simulink model "Lab_1b_sim"  (R2017a)
settings: Solver=VariableStepAuto  StartTime=0.0  StopTime=1.0  RelTol=1e-3
values from neighbouring files (symbols this model uses):
  alpha = 26.66    [Lab_1.m]    (also in Lab_2.m)
  alpha_p = 32.7345    [Lab_1.m]    (also in Lab_2.m)
  beta = 133.33    [Lab_1.m]    (also in Lab_2.m)
  K = f*(alpha_p.^2)/(4*beta)    [Lab_1.m]    (also in Lab_2.m)
  Kf = alpha_p/2    (= 16.36725)    [Lab_1.m]    (also in Lab_2.m)
settings Model: Creator=njohnson  LastModifiedBy=njohnson

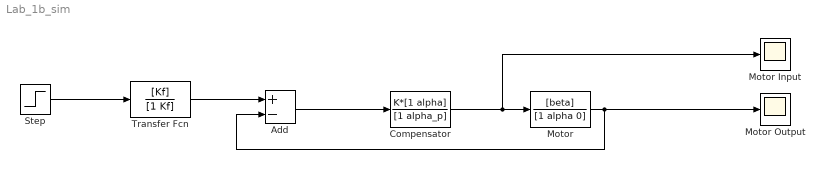
== system Lab_1b_sim ==
  Add : Sum  Inputs=+-
  "Compensator " : TransferFcn  Numerator=K*[1 alpha]  Denominator=[1 alpha_p]
  "Motor " : TransferFcn  Numerator=[beta]  Denominator=[1 alpha 0]
  Motor Input : Scope
  Motor Output : Scope
  Step : Step  Time=0  After=3  SampleTime=0
  Transfer Fcn : TransferFcn  Numerator=[Kf]  Denominator=[1 Kf]
  wires:
  Add/1 -> "Compensator "/1
  "Compensator "/1 -> Motor Input/1, "Motor "/1
  "Motor "/1 -> Motor Output/1, Add/2
  Step/1 -> Transfer Fcn/1
  Transfer Fcn/1 -> Add/1
